simulink model "Esempio"  (Simulink 8.3)
settings: Solver=FixedStepDiscrete  StartTime=0.0  StopTime=stopTimeSim  FixedStep=1  RelTol=1e-3
libraries: LibFactorGraph x13
settings Model: Creator=amedeobuonanno  LastModifiedBy=amedeobuonanno
settings OptimizationCC: ExpressionDepthLimit=2147483647
settings DebuggingCC: FcnCallInpInsideContextMsg=EnableAllAsWarning
settings GRTTargetCC: CombineOutputUpdateFcns=on  GRTInterface=off

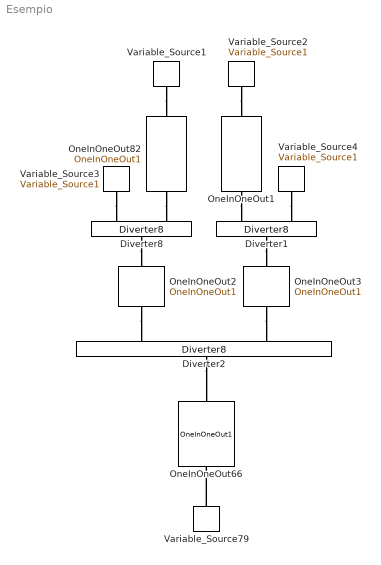
== system Esempio ==
  Diverter1 : LibFactorGraph/Diverter8  SystemSampleTime=-1
  Diverter2 : LibFactorGraph/Diverter8  SystemSampleTime=-1
  Diverter8 : LibFactorGraph/Diverter8  SystemSampleTime=-1
  OneInOneOut1 : LibFactorGraph/OneInOneOut1  var=1
  OneInOneOut2 : LibFactorGraph/OneInOneOut1  var=10
  OneInOneOut3 : LibFactorGraph/OneInOneOut1  var=11
  OneInOneOut66 : LibFactorGraph/OneInOneOut1  var=101
  OneInOneOut82 : LibFactorGraph/OneInOneOut1  var=0
  Variable_Source1 : LibFactorGraph/Variable_Source1  var=Atmp
  Variable_Source2 : LibFactorGraph/Variable_Source1  var=Stmp
  Variable_Source3 : LibFactorGraph/Variable_Source1  var=A
  Variable_Source4 : LibFactorGraph/Variable_Source1  var=S
  Variable_Source79 : LibFactorGraph/Variable_Source  var=C
  connections:
  Variable_Source79/LConn1 -- OneInOneOut66/LConn1
  Variable_Source1/LConn1 -- OneInOneOut82/RConn1
  Variable_Source2/LConn1 -- OneInOneOut1/RConn1
  OneInOneOut82/LConn1 -- Diverter8/LConn2
  OneInOneOut1/LConn1 -- Diverter1/LConn1
  Variable_Source3/LConn1 -- Diverter8/LConn1
  Variable_Source4/LConn1 -- Diverter1/LConn2
  Diverter8/RConn1 -- OneInOneOut2/RConn1
  Diverter1/RConn1 -- OneInOneOut3/RConn1
  OneInOneOut2/LConn1 -- Diverter2/LConn1
  OneInOneOut3/LConn1 -- Diverter2/LConn2
  Diverter2/RConn1 -- OneInOneOut66/RConn1
